simulink model "AOO_ver007_Serial"  (R2020a)
settings: Solver=FixedStepAuto  StartTime=0.0  StopTime=1  FixedStep=1e-3  RelTol=1e-3  EnableMultiTasking=on
undefined symbols (not defined in the file): D10, D11, D12, D2, D4, D5, D7, D8, D9, PTA0, PTA2, PTB23, PTB9, PTC3, PTC4, PTD0, PTD2, PTD3
libraries: frdmk64flib x14, etargetslib x3
settings Model: ExtModeTrigDuration=5  Creator=gigam  LastModifiedBy=Rahnn
settings OptimizationCC: EnhancedBackFolding=on  PassReuseOutputArgsAs=Individual arguments  ZeroExternalMemoryAtStartup=off  ZeroInternalMemoryAtStartup=off  MaxStackSize=64  OptimizeBlockOrder=speed  DifferentSizesBufferReuse=on  OptimizationCustomize=off  EfficientTunableParamExpr=on
settings DebuggingCC: ParameterTunabilityLossMsg=error
settings HardwareCC: ProdBitPerPointer=32  ProdBitPerSizeT=32  ProdBitPerPtrDiffT=32  ProdLargestAtomicInteger=Long  ProdLargestAtomicFloat=Double  ProdWordSize=32  ProdHWDeviceType=ARM Compatible->ARM Cortex
settings SFSimCC: MATLABDynamicMemAlloc=off
settings RTWCC: SystemTargetFile=ert.tlc  HardwareBoard=NXP FRDM-K64F  TemplateMakefile=ert_default_tmf  Toolchain=GNU Tools for ARM Embedded Processors
settings CodeAppCC: ForceParamTrailComments=on  IgnoreCustomStorageClasses=off  OperatorAnnotations=on  SimulinkDataObjDesc=on  SFDataObjDesc=on  InsertBlockDesc=on

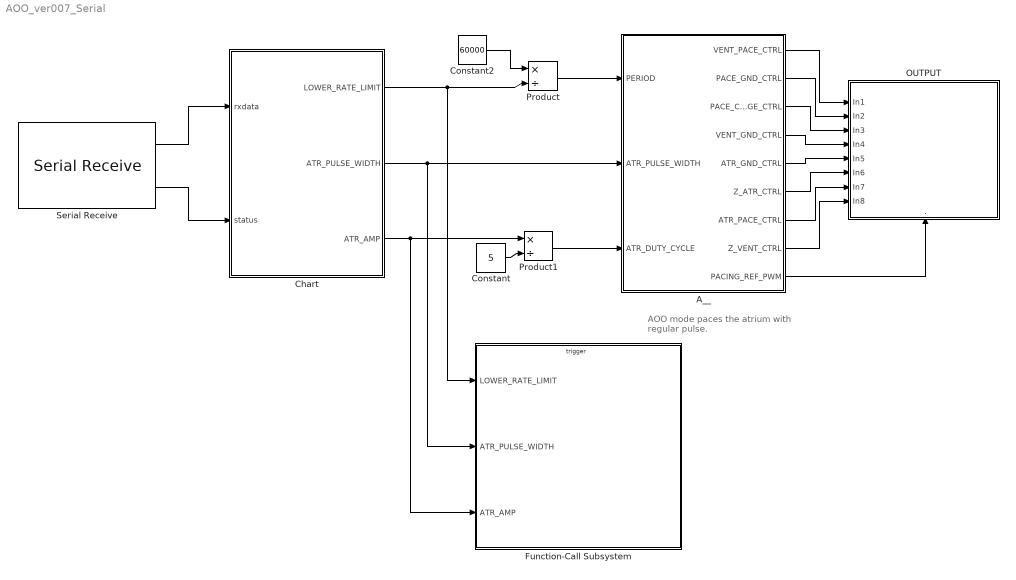
== system AOO_ver007_Serial ==
  note: AOO mode paces the atrium with regular pulse.
  A__ : Stateflow chart  TreatAsAtomicUnit=on
  Chart : Stateflow chart  TreatAsAtomicUnit=on
  Constant : Constant  Value=5
  Constant2 : Constant  Value=60000
  Function-Call Subsystem : Subsystem  TreatAsAtomicUnit=on
  OUTPUT : Subsystem
      settings: PortSchema="{\"entries\":[{\"content\":{\"sides\":[{\"content\":{\"connectorIds\":[\"In1\",\"In2\",\"In3\",\"In4\",\"In5\",\"In6\",\"In7\",\"In8\"]},\"type\":\"ConnectorPlacement.EquallySpacedRectSide\",\"uuid\":\"50e254ca-649e-457a-a1c0-3970395998e3\"},{\"content\":{\"connectorIds\":[],\"side\":\"RIGHT\"},\"type\":\"ConnectorPlacement.EquallySpacedRectSide\",\"uuid\":\"d7670675-e925-444e-9580-d2b53e4df198\"},{\"content\":{\"connectorIds\":[],\"side\":\"TOP\"},\"type\":\"ConnectorPlacement.EquallySpacedRectSide\",\"uuid\":\"432fabf6-6681-421d-882c-12b4d1ca9ae9\"},{\"content\":{\"connectorIds\":[\"In9\"],\"side\":\"BOTTOM\"},\"type\":\"ConnectorPlacement.EquallySpacedRectSide\",\"uuid\":\"b688b9eb-438e-4a02-9404-a817f809a45b\"}]},\"type\":\"ConnectorPlacement.EquallySpacedConnector\",\"uuid\":\"04b41c84-36c5-48e6-ac23-8c9a396cdfb3\"}],\"packageUris\":[\"http://schema.mathworks.com/mf0/Connector/19700101\"],\"version\":\"1.0\"}"
  Product : Product  Inputs=*/  OutDataTypeStr=uint16
  Product1 : Product  Inputs=*/
  Serial Receive : frdmk64flib/Serial Receive  SCIModule=0  Baudrate=uint32(9600)  Parity=None  StopBits=1  HardwareFlowControl=None  ByteOrder=LittleEndian  DataType=uint8  DataLength=14  BlockingMode=off  OutputStatus=on  SampleTime=-1
  wires:
  Product/1 -> A__/1(PERIOD)
  A__/1(VENT_PACE_CTRL) -> OUTPUT/1(In1)
  A__/2(PACE_GND_CTRL) -> OUTPUT/2(In2)
  A__/3(PACE_CHARGE_CTRL) -> OUTPUT/3(In3)
  A__/4(VENT_GND_CTRL) -> OUTPUT/4(In4)
  A__/5(ATR_GND_CTRL) -> OUTPUT/5(In5)
  A__/6(Z_ATR_CTRL) -> OUTPUT/6(In6)
  A__/7(ATR_PACE_CTRL) -> OUTPUT/7(In7)
  A__/8(Z_VENT_CTRL) -> OUTPUT/8(In8)
  Chart/2(ATR_PULSE_WIDTH) -> Function-Call Subsystem/2(ATR_PULSE_WIDTH), A__/2(ATR_PULSE_WIDTH)
  A__/9(PACING_REF_PWM) -> OUTPUT/9(.)
  Product1/1 -> A__/3(ATR_DUTY_CYCLE)
  Serial Receive/1 -> Chart/1(rxdata)
  Serial Receive/2 -> Chart/2(status)
  Chart/1(LOWER_RATE_LIMIT) -> Function-Call Subsystem/1(LOWER_RATE_LIMIT), Product/2
  Constant2/1 -> Product/1
  Chart/3(ATR_AMP) -> Function-Call Subsystem/3(ATR_AMP), Product1/1
  Constant/1 -> Product1/2

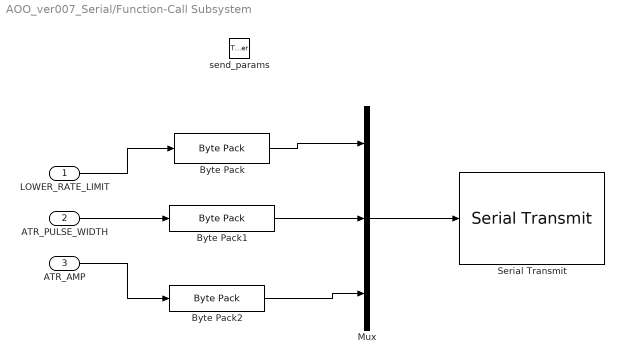
== system AOO_ver007_Serial/Function-Call Subsystem ==
  LOWER_RATE_LIMIT : Inport  OutDataTypeStr=uint16
  ATR_PULSE_WIDTH : Inport  Port=2  OutDataTypeStr=uint16
  ATR_AMP : Inport  Port=3  OutDataTypeStr=double
  send_params : TriggerPort  TriggerType=function-call  IsSimulinkFunction=on  FunctionName=send_params  VariantControl=Variant
  Byte Pack : etargetslib/Byte Pack  datatypes={'uint16'}  byteAlign=1
  Byte Pack1 : etargetslib/Byte Pack  datatypes={'uint16'}  byteAlign=1
  Byte Pack2 : etargetslib/Byte Pack  datatypes={'double'}  byteAlign=1
  Mux : Mux  Inputs=3
  Serial Transmit : frdmk64flib/Serial Transmit  SCIModule=0  Baudrate=uint32(9600)  Parity=None  StopBits=1  HardwareFlowControl=None  ByteOrder=LittleEndian  BlockingMode=on  OutputStatus=off
  wires:
  LOWER_RATE_LIMIT/1 -> Byte Pack/1
  Byte Pack/1 -> Mux/1
  ATR_PULSE_WIDTH/1 -> Byte Pack1/1
  Byte Pack1/1 -> Mux/2
  ATR_AMP/1 -> Byte Pack2/1
  Byte Pack2/1 -> Mux/3
  Mux/1 -> Serial Transmit/1

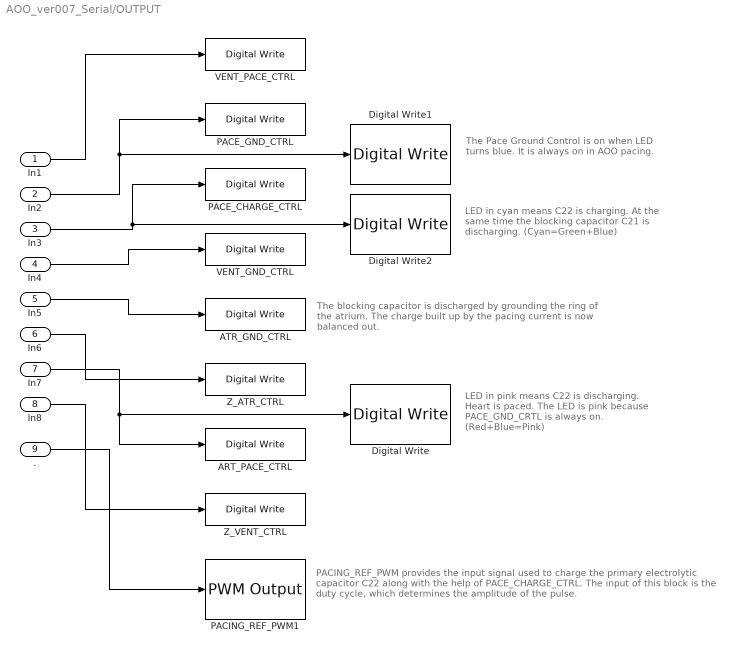
== system AOO_ver007_Serial/OUTPUT ==
  note: The blocking capacitor is discharged by grounding the ring of the atrium. The charge built up by the pacing current is now balanced out.
  note: LED in pink means C22 is discharging. Heart is paced. The LED is pink because PACE_GND_CRTL is always on. (Red+Blue=Pink)
  note: The Pace Ground Control is on when LED turns blue. It is always on in AOO pacing.
  note: LED in cyan means C22 is charging. At the same time the blocking capacitor C21 is discharging. (Cyan=Green+Blue)
  note: PACING_REF_PWM provides the input signal used to charge the primary electrolytic capacitor C22 along with the help of PACE_CHARGE_CTRL. The input of this block is the duty cycle, which determines the amplitude of the pulse.
  In1 : Inport
  In2 : Inport  Port=2
  In3 : Inport  Port=3
  In4 : Inport  Port=4
  In5 : Inport  Port=5
  In6 : Inport  Port=6
  In7 : Inport  Port=7
  In8 : Inport  Port=8
  . : Inport  Port=9
  ART_PACE_CTRL : frdmk64flib/Digital Write  Whichpin=PTA0 (D8)
  ATR_GND_CTRL : frdmk64flib/Digital Write  Whichpin=PTD2 (D11)
  Digital Write : frdmk64flib/Digital Write  Whichpin=RED_LED
  Digital Write1 : frdmk64flib/Digital Write  Whichpin=BLUE_LED
  Digital Write2 : frdmk64flib/Digital Write  Whichpin=GREEN_LED
  PACE_CHARGE_CTRL : frdmk64flib/Digital Write  Whichpin=PTB9 (D2)
  PACE_GND_CTRL : frdmk64flib/Digital Write  Whichpin=PTD0 (D10)
  PACING_REF_PWM1 : frdmk64flib/PWM Output  Whichpin=PTA2 (D5)  InitialFrequency=2000  InitialDutyCycle=100
  VENT_GND_CTRL : frdmk64flib/Digital Write  Whichpin=PTD3 (D12)
  VENT_PACE_CTRL : frdmk64flib/Digital Write  Whichpin=PTC4 (D9)
  Z_ATR_CTRL : frdmk64flib/Digital Write  Whichpin=PTB23 (D4)
  Z_VENT_CTRL : frdmk64flib/Digital Write  Whichpin=PTC3 (D7)
  wires:
  In7/1 -> Digital Write/1, ART_PACE_CTRL/1
  In6/1 -> Z_ATR_CTRL/1
  In3/1 -> PACE_CHARGE_CTRL/1, Digital Write2/1
  In5/1 -> ATR_GND_CTRL/1
  In2/1 -> PACE_GND_CTRL/1, Digital Write1/1
  In1/1 -> VENT_PACE_CTRL/1
  In4/1 -> VENT_GND_CTRL/1
  In8/1 -> Z_VENT_CTRL/1
  ./1 -> PACING_REF_PWM1/1

== stateflow chart AOO_ver007_Serial/Chart ==
  state SET_PARAM
    entry:
    LOWER_RATE_LIMIT = typecast(rxdata(3:4),'uint16');
    ATR_PULSE_WIDTH = typecast(rxdata(5:6),'uint16');
    ATR_AMP = typecast(rxdata(7:14),'double');
  state INITIAL
    %Set the initial values of paprameters
    entry:
    LOWER_RATE_LIMIT = 60;
    ATR_PULSE_WIDTH = 10;
    ATR_AMP = 4;
  state STANDBY
    %Waiting for COM
  state ECHO_PARAM
    %Sends back the currrent value of the parameters
    entry:
    send_params();
  SET_PARAM -> STANDBY
  (default) -> INITIAL
  (junction 9) -> SET_PARAM [order 1] : [rxdata(2)==hex2dec('55')]
  (junction 7) -> STANDBY [order 2]
  INITIAL -> STANDBY
  STANDBY -> (junction 7) : [status==0]
  (junction 7) -> (junction 9) [order 1] : [rxdata(1)==hex2dec('16')]
  (junction 9) -> ECHO_PARAM [order 2] : [rxdata(2)==hex2dec('22')]
  ECHO_PARAM -> STANDBY
  data: rxdata input uint8; status input uint8; LOWER_RATE_LIMIT output uint16; ATR_PULSE_WIDTH output uint16; ATR_AMP output double

== stateflow chart AOO_ver007_Serial/A__ ==
  state Pace
    entry:
    PACE_CHARGE_CTRL = false;
    PACE_GND_CTRL = true;
    VENT_PACE_CTRL = false;
    VENT_GND_CTRL = false;
    Z_VENT_CTRL = false;
    Z_ATR_CTRL = false;
    ATR_GND_CTRL = false;
    ATR_PACE_CTRL = true;
    %C22 Discharge -> Pace Atrium -> C21 Saturated
  state Charge
    entry:
    PACE_GND_CTRL = true;
    ATR_PACE_CTRL = false;
    Z_VENT_CTRL = false;
    Z_ATR_CTRL = false;
    VENT_GND_CTRL = false;
    ATR_GND_CTRL = true;
    %Discharging C21
    VENT_PACE_CTRL = false;
    ATR_PACE_CTRL = false;
    PACING_REF_PWM = ATR_DUTY_CYCLE;
    PACE_CHARGE_CTRL = true;
    %Charging Primary Capacitor (C22)
  (default) -> Charge
  Charge -> Pace : [after(PERIOD-ATR_PULSE_WIDTH,msec)]
  Pace -> Charge : [after(ATR_PULSE_WIDTH,msec)]
  data: VENT_PACE_CTRL output boolean; PACE_GND_CTRL output boolean; PACE_CHARGE_CTRL output boolean; VENT_GND_CTRL output boolean; ATR_GND_CTRL output boolean; Z_ATR_CTRL output boolean; ATR_PACE_CTRL output boolean; Z_VENT_CTRL output boolean; PERIOD input uint16; ATR_PULSE_WIDTH input uint16; ATR_DUTY_CYCLE input double; PACING_REF_PWM output double
